simulink model "parallel_simulink_MOO_GSTA"  (R2018b)
settings: Solver=FixedStepAuto  StartTime=0.0  StopTime=42  FixedStep=0.005  RelTol=1e-3
InitFcn:
  | parameters_initial
model workspace: external: MAT-File (data not in the file)
values from neighbouring files (symbols this model uses):
  v0 = 0    [parameters_initial.m]
  x0 = 0.1    [parameters_initial.m]    (also in x0.mat = [19.4118556352 7.3849356224 17.7302386615 16.3509418416 10.3)
  x_pareto = [13.7929   10.4417    0.1921    0.0962]    [parameters_initial.m]
libraries: sdolib x1
settings Model: Creator=DING  LastModifiedBy=DNN
settings SolverCC: ZeroCrossAlgorithm=Adaptive
settings OptimizationCC: DefaultParameterBehavior=Inlined  EnhancedBackFolding=on  PassReuseOutputArgsAs=Individual arguments  MaxStackSize=64  OptimizeBlockOrder=speed  DifferentSizesBufferReuse=on  OptimizationCustomize=off
settings DebuggingCC: IgnoredZcDiagnostic=none  ParameterTunabilityLossMsg=error
settings HardwareCC: ProdBitPerPointer=32  ProdBitPerSizeT=32  ProdBitPerPtrDiffT=32  ProdLargestAtomicInteger=Long  ProdLargestAtomicFloat=Double  ProdWordSize=32  ProdHWDeviceType=ARM Compatible->ARM 11
settings SFSimCC: MATLABDynamicMemAlloc=off
settings RTWCC: SystemTargetFile=ert.tlc  TemplateMakefile=ert_default_tmf  GenerateReport=on  Toolchain=Catkin  IncludeHyperlinkInReport=on  LaunchReport=on  GenerateTraceInfo=on  GenerateTraceReport=on  GenerateTraceReportSl=on  GenerateTraceReportSf=on  GenerateTraceReportEml=on
settings CodeAppCC: ForceParamTrailComments=on  IgnoreCustomStorageClasses=off  OperatorAnnotations=on  SimulinkDataObjDesc=on  SFDataObjDesc=on  InsertBlockDesc=on
settings ERTTargetCC: ERTCustomFileTemplate=example_file_process.tlc

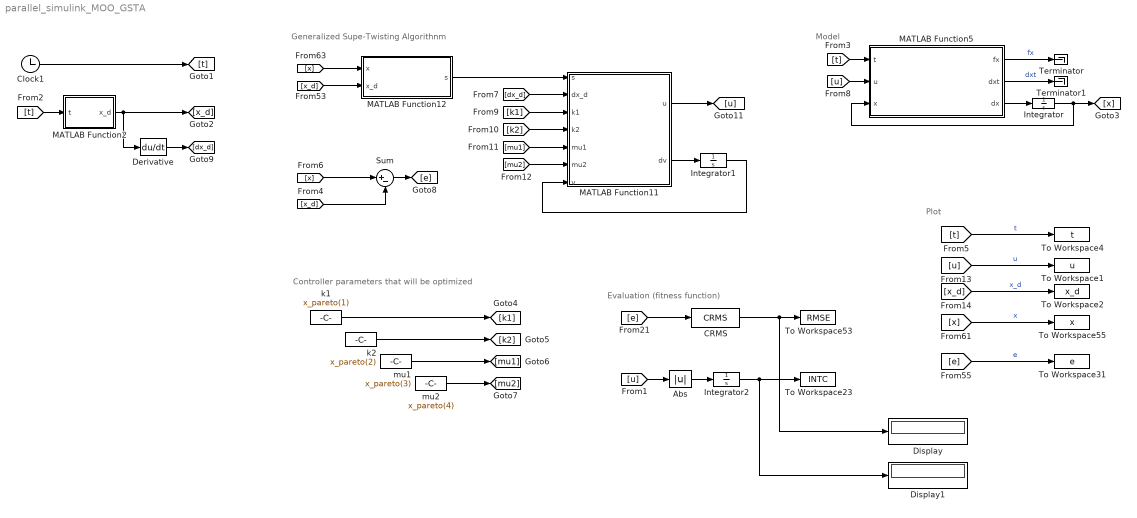
== system parallel_simulink_MOO_GSTA ==
  note: Plot
  note: Model
  note: Evaluation (fitness function)
  note: Controller parameters that will be optimized
  note: Generalized Supe-Twisting Algorithnm
  Abs : Abs
  CRMS : sdolib/RMS Blocks/CRMS
      settings: SourceProductName=Simulink Design Optimization  SourceProductBaseCode=SO
  Clock1 : Clock
  Derivative : Derivative
  Display : Display
  Display1 : Display
  Integrator : Integrator  InitialCondition=x0
  Integrator1 : Integrator  InitialCondition=v0
  Integrator2 : Integrator  InitialCondition=v0
  MATLAB Function11 : MATLAB Function  TreatAsAtomicUnit=on
  MATLAB Function12 : MATLAB Function  TreatAsAtomicUnit=on
  MATLAB Function2 : MATLAB Function  TreatAsAtomicUnit=on
  MATLAB Function5 : MATLAB Function  TreatAsAtomicUnit=on
  Sum : Sum  Inputs=|+-
  Terminator : Terminator
  Terminator1 : Terminator
  To Workspace1 : ToWorkspace  VariableName=u  SampleTime=-1
  To Workspace2 : ToWorkspace  VariableName=x_d  SampleTime=-1
  To Workspace23 : ToWorkspace  VariableName=INTC  SampleTime=-1
      settings: MaxDataPoints=1
  To Workspace31 : ToWorkspace  VariableName=e  SampleTime=-1
  To Workspace4 : ToWorkspace  VariableName=t  SampleTime=-1
  To Workspace53 : ToWorkspace  VariableName=RMSE  SampleTime=-1
      settings: MaxDataPoints=1
  To Workspace55 : ToWorkspace  VariableName=x  SampleTime=-1
  k1 : Constant  Value=x_pareto(1)
  k2 : Constant  Value=x_pareto(2)
  mu1 : Constant  Value=x_pareto(3)
  mu2 : Constant  Value=x_pareto(4)
  wires:
  CRMS/1 -> To Workspace53/1, Display/1
  mu1/1 -> [mu1]
  k2/1 -> [k2]
  mu2/1 -> [mu2]
  k1/1 -> [k1]
  [x_d] -> MATLAB Function12/2(x_d)
  MATLAB Function11/1(u) -> [u]
  MATLAB Function12/1(s) -> MATLAB Function11/1(s)
  [x] -> MATLAB Function12/1(x)
  [t] -> To Workspace4/1  "t"
  [x] -> To Workspace55/1  "x"
  [e] -> To Workspace31/1  "e"
  MATLAB Function5/3(dx) -> Integrator/1
  Integrator/1 -> [x], MATLAB Function5/3(x)
  [t] -> MATLAB Function5/1(t)
  [u] -> MATLAB Function5/2(u)
  MATLAB Function2/1(x_d) -> [x_d], Derivative/1
  [k1] -> MATLAB Function11/3(k1)
  [k2] -> MATLAB Function11/4(k2)
  [mu1] -> MATLAB Function11/5(mu1)
  [mu2] -> MATLAB Function11/6(mu2)
  MATLAB Function11/2(dv) -> Integrator1/1
  Integrator1/1 -> MATLAB Function11/7(v)
  [e] -> CRMS/1
  [u] -> Abs/1
  Integrator2/1 -> To Workspace23/1, Display1/1
  Clock1/1 -> [t]
  [t] -> MATLAB Function2/1(t)
  [x] -> Sum/1
  [x_d] -> Sum/2
  Sum/1 -> [e]
  Derivative/1 -> [dx_d]
  [dx_d] -> MATLAB Function11/2(dx_d)
  [u] -> To Workspace1/1  "u"
  [x_d] -> To Workspace2/1  "x_d"
  MATLAB Function5/1(fx) -> Terminator/1  "fx"
  MATLAB Function5/2(dxt) -> Terminator1/1  "dxt"
  Abs/1 -> Integrator2/1

== matlab function parallel_simulink_MOO_GSTA/MATLAB Function2 ==
  data: x_d output; t input
function x_d= desired(t)

x_d=sin(0.8*t)+cos(t);

end

== matlab function parallel_simulink_MOO_GSTA/MATLAB Function5 ==
  data: fx output; dxt output; dx output; t input; u input; x input
function [fx,dxt,dx]= Model(t,u,x)

fx=0.6*sin(x)+0.7*x^2-1.5*x;
dxt=0.8*cos(x)*x+0.05*cos(3*t)+0.08*sin(t);
dx=fx+dxt+u;

end

== matlab function parallel_simulink_MOO_GSTA/MATLAB Function11 ==
  data: s input; dx_d input; u output; dv output; k1 input; k2 input; mu1 input; mu2 input; v input
function [u,dv] = GSTA(s,dx_d,k1,k2,mu1,mu2,v)

fa_1s=mu1*abs(s)^0.5*sign(s)+mu2*s;
fa_2s=0.5*mu1^2*sign(s)+1.5*mu1*mu2*abs(s)^0.5*sign(s)+mu2^2*s;
dv=-k2*fa_2s;
u=dx_d-k1*fa_1s+v;

end

== matlab function parallel_simulink_MOO_GSTA/MATLAB Function12 ==
  data: x input; x_d input; s output
function s = sliding_face(x,x_d)

s=x-x_d;

end
